simulink library "lib_EMachine_2017a"  (R2017b)
settings: Solver=VariableStepAuto  StartTime=0.0  StopTime=10.0  RelTol=1e-3
undefined symbols (not defined in the file): EngineTorqueReal, mot, motor_Trq, t_amb, time, tloop
libraries: simulink x5, autolibmappedmotor x3
(part 3 of 3)

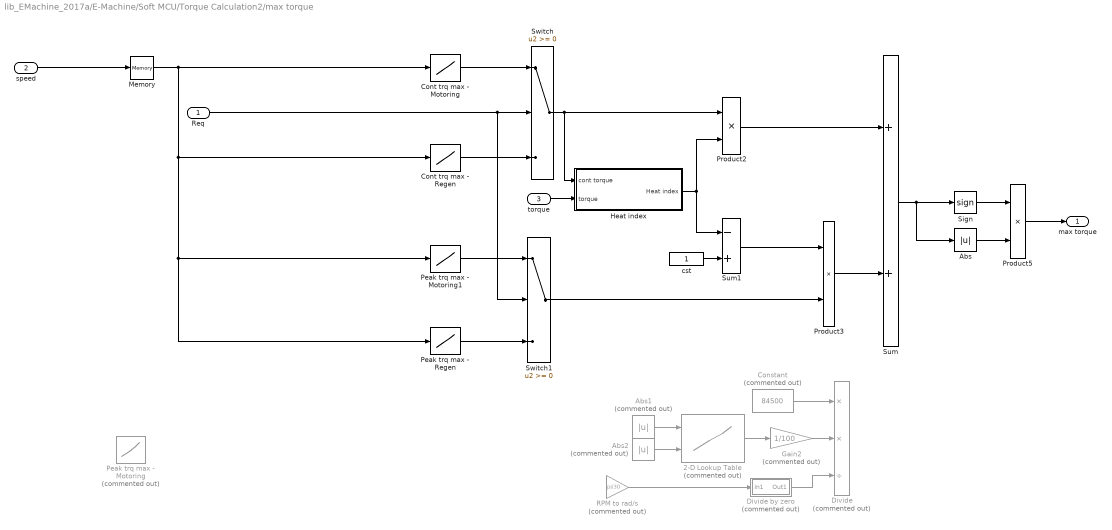
== system lib_EMachine_2017a/E-Machine/Soft MCU/Torque Calculation2/max torque  ==
  Req : Inport
  speed : Inport  Port=2
  torque : Inport  Port=3
  2-D Lookup Table : Lookup_n-D  Commented=on  BreakpointsForDimension1=mot.plant.init.eff_trq.idx2_trq  BreakpointsForDimension2=mot.plant.init.eff_trq.idx1_spd  Table=mot.plant.init.eff_trq.map  InternalRulePriority=Speed  RndMeth=Simplest  InputSameDT=on
  Abs : Abs  SaturateOnIntegerOverflow=on
  Abs1 : Abs  Commented=on
  Abs2 : Abs  Commented=on
  Constant : Constant  Commented=on  Value=84500
  Cont trq max - Motoring : Lookup  InputValues=mot.plant.init.motor.trq_cont.idx1_spd  Table=mot.plant.init.motor.trq_cont.map  LookUpMeth=Interpolation-Use End Values  SaturateOnIntegerOverflow=on
  Cont trq max - Regen : Lookup  InputValues=mot.plant.init.regen.trq_cont.idx1_spd  Table=mot.plant.init.regen.trq_cont.map  LookUpMeth=Interpolation-Use End Values  SaturateOnIntegerOverflow=on
  Divide : Product  Commented=on  Inputs=**/
  Divide by zero : Subsystem  Commented=on
  Gain2 : Gain  Commented=on  Gain=1/100
  Heat index : Subsystem
  Memory : Memory
  Peak trq max - Motoring : Lookup  Commented=on  InputValues=mot.plant.init.regen.trq_max.idx1_spd  Table=mot.plant.init.motor.trq_max.map  LookUpMeth=Interpolation-Use End Values  SaturateOnIntegerOverflow=on
  Peak trq max - Motoring1 : Lookup  InputValues=mot.plant.init.regen.trq_max.idx1_spd  Table=mot.plant.init.motor.trq_max.map  LookUpMeth=Interpolation-Use End Values  SaturateOnIntegerOverflow=on
  Peak trq max - Regen : Lookup  InputValues=mot.plant.init.regen.trq_max.idx1_spd  Table=mot.plant.init.regen.trq_max.map  LookUpMeth=Interpolation-Use End Values  SaturateOnIntegerOverflow=on
  Product2 : Product  SaturateOnIntegerOverflow=on  InputSameDT=on  OutDataTypeStr=Inherit: Same as first input
  Product3 : Product  SaturateOnIntegerOverflow=on  InputSameDT=on  OutDataTypeStr=Inherit: Same as first input
  Product5 : Product  SaturateOnIntegerOverflow=on  InputSameDT=on  OutDataTypeStr=Inherit: Same as first input
  RPM to rad/s : Gain  Commented=on  Gain=pi/30
  Sign : Signum
  Sum : Sum  SaturateOnIntegerOverflow=on  InputSameDT=on  OutDataTypeStr=Inherit: Same as first input
  Sum1 : Sum  Inputs=-+  SaturateOnIntegerOverflow=on  InputSameDT=on  OutDataTypeStr=Inherit: Same as first input
  Switch : Switch  SaturateOnIntegerOverflow=on
  Switch1 : Switch  SaturateOnIntegerOverflow=on
  cst : Constant
  max torque : Outport
  wires:
  Peak trq max - Motoring1/1 -> Switch1/1
  Divide by zero/1(Out1) -> Divide/3
  Req/1 -> Switch1/2, Switch/2
  Gain2/1 -> Divide/2
  2-D Lookup Table/1 -> Gain2/1
  Abs1/1 -> 2-D Lookup Table/1
  Abs2/1 -> 2-D Lookup Table/2
  RPM to rad/s/1 -> Divide by zero/1(In1)
  Constant/1 -> Divide/1
  speed/1 -> Memory/1
  Memory/1 -> Peak trq max - Regen/1, Peak trq max - Motoring1/1, Cont trq max - Regen/1, Cont trq max - Motoring/1
  Sign/1 -> Product5/1
  Product5/1 -> max torque/1
  Sum/1 -> Sign/1, Abs/1
  Abs/1 -> Product5/2
  torque/1 -> Heat index/2(torque)
  Cont trq max - Motoring/1 -> Switch/1
  Cont trq max - Regen/1 -> Switch/3
  Peak trq max - Regen/1 -> Switch1/3
  Switch/1 -> Product2/1, Heat index/1(cont torque)
  Switch1/1 -> Product3/2
  Product2/1 -> Sum/1
  Sum1/1 -> Product3/1
  Product3/1 -> Sum/2
  cst/1 -> Sum1/2
  Heat index/1(Heat index) -> Sum1/1, Product2/2

== system lib_EMachine_2017a/E-Machine/Soft MCU/Torque Calculation3/Subsystem ==
  In1 : Inport
  In2 : Inport  Port=2
  In3 : Inport  Port=3
  Switch : Switch  Criteria=u2 > Threshold  ZeroCross=off
  Torq : Outport
  wires:
  Switch/1 -> Torq/1
  In1/1 -> Switch/1
  In3/1 -> Switch/3
  In2/1 -> Switch/2

== system lib_EMachine_2017a/E-Machine/Soft MCU/Torque Calculation3/Subsystem1 ==
  In1 : Inport
  In2 : Inport  Port=2
  In3 : Inport  Port=3
  Switch : Switch  Criteria=u2 > Threshold  ZeroCross=off
  Current : Outport
  wires:
  In2/1 -> Switch/2
  In3/1 -> Switch/3
  In1/1 -> Switch/1
  Switch/1 -> Current/1

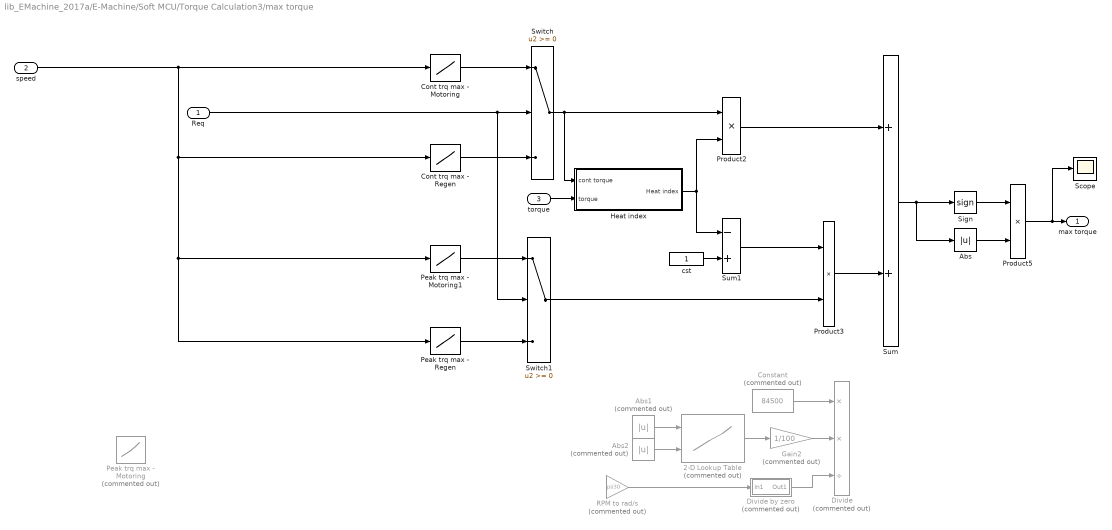
== system lib_EMachine_2017a/E-Machine/Soft MCU/Torque Calculation3/max torque  ==
  Req : Inport
  speed : Inport  Port=2
  torque : Inport  Port=3
  2-D Lookup Table : Lookup_n-D  Commented=on  BreakpointsForDimension1=mot.plant.init.eff_trq.idx2_trq  BreakpointsForDimension2=mot.plant.init.eff_trq.idx1_spd  Table=mot.plant.init.eff_trq.map  InternalRulePriority=Speed  RndMeth=Simplest  InputSameDT=on
  Abs : Abs  ZeroCross=off  SaturateOnIntegerOverflow=on
  Abs1 : Abs  Commented=on
  Abs2 : Abs  Commented=on
  Constant : Constant  Commented=on  Value=84500
  Cont trq max - Motoring : Lookup  InputValues=mot.plant.init.motor.trq_cont.idx1_spd  Table=mot.plant.init.motor.trq_cont.map  LookUpMeth=Interpolation-Use End Values  SaturateOnIntegerOverflow=on
  Cont trq max - Regen : Lookup  InputValues=mot.plant.init.regen.trq_cont.idx1_spd  Table=mot.plant.init.regen.trq_cont.map  LookUpMeth=Interpolation-Use End Values  SaturateOnIntegerOverflow=on
  Divide : Product  Commented=on  Inputs=**/
  Divide by zero : Subsystem  Commented=on
  Gain2 : Gain  Commented=on  Gain=1/100
  Heat index : Subsystem
  Peak trq max - Motoring : Lookup  Commented=on  InputValues=mot.plant.init.regen.trq_max.idx1_spd  Table=mot.plant.init.motor.trq_max.map  LookUpMeth=Interpolation-Use End Values  SaturateOnIntegerOverflow=on
  Peak trq max - Motoring1 : Lookup  InputValues=mot.plant.init.regen.trq_max.idx1_spd  Table=mot.plant.init.motor.trq_max.map  LookUpMeth=Interpolation-Use End Values  SaturateOnIntegerOverflow=on
  Peak trq max - Regen : Lookup  InputValues=mot.plant.init.regen.trq_max.idx1_spd  Table=mot.plant.init.regen.trq_max.map  LookUpMeth=Interpolation-Use End Values  SaturateOnIntegerOverflow=on
  Product2 : Product  SaturateOnIntegerOverflow=on  InputSameDT=on  OutDataTypeStr=Inherit: Same as first input
  Product3 : Product  SaturateOnIntegerOverflow=on  InputSameDT=on  OutDataTypeStr=Inherit: Same as first input
  Product5 : Product  SaturateOnIntegerOverflow=on  InputSameDT=on  OutDataTypeStr=Inherit: Same as first input
  RPM to rad/s : Gain  Commented=on  Gain=pi/30
  Scope : Scope
  Sign : Signum  ZeroCross=off
  Sum : Sum  SaturateOnIntegerOverflow=on  InputSameDT=on  OutDataTypeStr=Inherit: Same as first input
  Sum1 : Sum  Inputs=-+  SaturateOnIntegerOverflow=on  InputSameDT=on  OutDataTypeStr=Inherit: Same as first input
  Switch : Switch  SaturateOnIntegerOverflow=on
  Switch1 : Switch  SaturateOnIntegerOverflow=on
  cst : Constant
  max torque : Outport
  wires:
  Peak trq max - Motoring1/1 -> Switch1/1
  Divide by zero/1(Out1) -> Divide/3
  Req/1 -> Switch1/2, Switch/2
  Gain2/1 -> Divide/2
  2-D Lookup Table/1 -> Gain2/1
  Abs1/1 -> 2-D Lookup Table/1
  Abs2/1 -> 2-D Lookup Table/2
  RPM to rad/s/1 -> Divide by zero/1(In1)
  Constant/1 -> Divide/1
  speed/1 -> Peak trq max - Regen/1, Peak trq max - Motoring1/1, Cont trq max - Regen/1, Cont trq max - Motoring/1
  Sign/1 -> Product5/1
  Product5/1 -> max torque/1, Scope/1
  Sum/1 -> Sign/1, Abs/1
  Abs/1 -> Product5/2
  torque/1 -> Heat index/2(torque)
  Cont trq max - Motoring/1 -> Switch/1
  Cont trq max - Regen/1 -> Switch/3
  Peak trq max - Regen/1 -> Switch1/3
  Switch/1 -> Product2/1, Heat index/1(cont torque)
  Switch1/1 -> Product3/2
  Product2/1 -> Sum/1
  Sum1/1 -> Product3/1
  Product3/1 -> Sum/2
  cst/1 -> Sum1/2
  Heat index/1(Heat index) -> Sum1/1, Product2/2

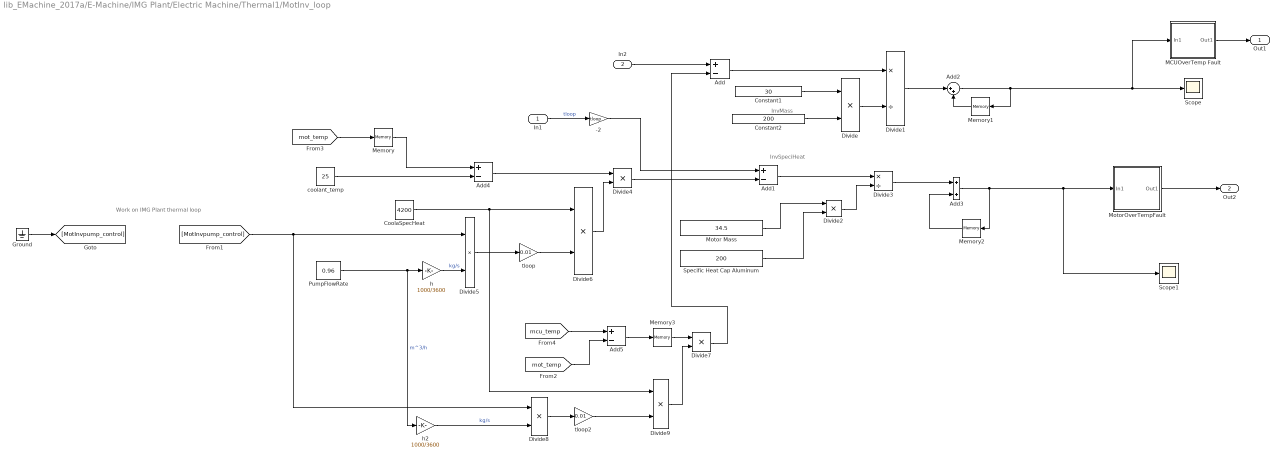
== system lib_EMachine_2017a/E-Machine/IMG Plant/Electric Machine/Thermal1/MotInv_loop ==
  note: InvSpeciHeat
  note: InvMass
  note: Work on IMG Plant thermal loop
  In1 : Inport
  In2 : Inport  Port=2
  -2 : Gain  Gain=tloop
  Add{,1,4..5} (4 alike) : Sum  Inputs=+-
  Add2 : Sum  Inputs=|++
  Add3 : Sum
  Constant1 : Constant  Value=30
  Constant2 : Constant  Value=200
  CoolaSpecHeat : Constant  Value=4200
  Divide{,2,4..9} (8 alike) : Product  Inputs=**
  Divide1 : Product  Inputs=*/
  Divide3 : Product  Inputs=*/
  Ground : Ground
  MCUOverTemp Fault : Subsystem
  Memory : Memory
  Memory1 : Memory  InitialCondition=25
  Memory2 : Memory  InitialCondition=25
  Memory3 : Memory
  Motor Mass : Constant  Value=34.5
  MotorOverTempFault : Subsystem
  PumpFlowRate : Constant  Value=0.96
  Scope : Scope
  Scope1 : Scope
  Specific Heat Cap Aluminum : Constant  Value=200
  coolant_temp : Constant  Value=25
  h : Gain  Gain=1000/3600
  h2 : Gain  Gain=1000/3600
  tloop : Gain  Gain=0.01
  tloop2 : Gain  Gain=0.01
  Out1 : Outport
  Out2 : Outport  Port=2
  wires:
  Ground/1 -> [MotInvpump_control]
  Memory/1 -> Add4/1
  Add1/1 -> Divide3/1
  Memory1/1 -> Add2/2
  coolant_temp/1 -> Add4/2
  Divide/1 -> Divide1/2
  Specific Heat Cap Aluminum/1 -> Divide2/2
  Constant1/1 -> Divide/1
  Add/1 -> Divide1/1
  Memory2/1 -> Add3/2
  Add4/1 -> Divide4/1
  Add3/1 -> Scope1/1, MotorOverTempFault/1(In1), Memory2/1
  Divide6/1 -> Divide4/2
  Divide3/1 -> Add3/1
  Divide5/1 -> tloop/1
  Add2/1 -> MCUOverTemp Fault/1(In1), Scope/1, Memory1/1
  Divide2/1 -> Divide3/2
  Constant2/1 -> Divide/2
  Motor Mass/1 -> Divide2/1
  Divide1/1 -> Add2/1
  Divide7/1 -> Add/2
  h/1 -> Divide5/2  "kg/s"
  tloop/1 -> Divide6/2
  CoolaSpecHeat/1 -> Divide6/1, Divide9/1
  PumpFlowRate/1 -> h/1, h2/1  "m^3/h"
  h2/1 -> Divide8/2  "kg/s"
  Divide9/1 -> Divide7/2
  Divide8/1 -> tloop2/1
  tloop2/1 -> Divide9/2
  Divide4/1 -> Add1/2
  Add5/1 -> Memory3/1
  Memory3/1 -> Divide7/1
  MCUOverTemp Fault/1(Out1) -> Out1/1
  MotorOverTempFault/1(Out1) -> Out2/1
  [mot_temp] -> Memory/1
  [mcu_temp] -> Add5/1
  [mot_temp] -> Add5/2
  In1/1 -> -2/1  "tloop"
  In2/1 -> Add/1
  -2/1 -> Add1/1
  [MotInvpump_control] -> Divide5/1, Divide8/1

== system lib_EMachine_2017a/E-Machine/IMG Plant/Electric Machine/Thermal1/Motor Thermal ==
  In1 : Inport
  Add1 : Sum  Inputs=+-
  Add2 : Sum
  Divide : Product  Inputs=*/
  Lower Limit : Subsystem  mask{Lolimit=t_amb+20}
      mask prompts: Lolimit "Lower Limit"
  Memory1 : Memory
  Motor Mass : Constant  Value=mot.plant.init.motor_mass
  Product : Product  RndMeth=Zero
  "Pump " : Constant  Value=0
  Specific Heat Cap Aluminum : Constant  Value=mot.plant.init.specific_heat
  tloop : Gain  Gain=tloop
  Out1 : Outport
  wires:
  Specific Heat Cap Aluminum/1 -> Product/2  "J/kg*K"
  Product/1 -> Divide/2
  Memory1/1 -> Add2/2
  Add2/1 -> Lower Limit/1(In1)
  Lower Limit/1(Out1) -> Out1/1, Memory1/1
  Divide/1 -> Add2/1
  tloop/1 -> Divide/1  "J"
  Motor Mass/1 -> Product/1  "kg"
  "Pump "/1 -> Add1/2
  In1/1 -> Add1/1
  Add1/1 -> tloop/1

== system lib_EMachine_2017a/E-Machine/IMG Plant/Electric Machine/Torque Calculation1/max torque  ==
  cmd : Inport
  speed : Inport  Port=2
  Memory : Memory
  Peak trq max - Motoring : Lookup  InputValues=mot.plant.init.regen.trq_max.idx1_spd  Table=mot.plant.init.motor.trq_max.map  LookUpMeth=Interpolation-Use End Values  SaturateOnIntegerOverflow=on
  Peak trq max - Regen : Lookup  InputValues=mot.plant.init.regen.trq_max.idx1_spd  Table=mot.plant.init.regen.trq_max.map  LookUpMeth=Interpolation-Use End Values  SaturateOnIntegerOverflow=on
  Switch1 : Switch  SaturateOnIntegerOverflow=on
  rad/s  to RPM : Gain  Gain=30/pi
  max torque : Outport
  wires:
  Peak trq max - Motoring/1 -> Switch1/1
  speed/1 -> rad/s  to RPM/1
  cmd/1 -> Switch1/2
  Switch1/1 -> max torque/1
  Memory/1 -> Peak trq max - Motoring/1, Peak trq max - Regen/1
  rad/s  to RPM/1 -> Memory/1
  Peak trq max - Regen/1 -> Switch1/3

== system lib_EMachine_2017a/E-Machine/IMG Plant2/Thermal/Motor Thermal/Lower Limit ==
  In1 : Inport
  Constant3 : Constant  Value=Lolimit
  MinMax : MinMax  Function=max  Inputs=2
  Out1 : Outport
  wires:
  In1/1 -> MinMax/1
  Constant3/1 -> MinMax/2
  MinMax/1 -> Out1/1

== system lib_EMachine_2017a/E-Machine/IMG Plant2/Thermal1/MotInv_loop/MCUOverTemp Fault ==
  In1 : Inport
  Gain : Gain  Gain=3
  Switch : Switch  Threshold=1
  Out1 : Outport
  wires:
  In1/1 -> Switch/3, Gain/1
  [MCUOverTemp] -> Switch/2
  Gain/1 -> Switch/1
  Switch/1 -> Out1/1

== system lib_EMachine_2017a/E-Machine/IMG Plant2/Thermal1/MotInv_loop/MotorOverTempFault ==
  In1 : Inport
  Gain : Gain  Gain=2
  Switch1 : Switch  Threshold=1
  Out1 : Outport
  wires:
  In1/1 -> Gain/1, Switch1/3
  [MotOverTemp] -> Switch1/2
  Gain/1 -> Switch1/1
  Switch1/1 -> Out1/1

== system lib_EMachine_2017a/E-Machine/IMG Plant2/Thermal1/Motor Thermal/Lower Limit ==
  In1 : Inport
  Constant3 : Constant  Value=Lolimit
  MinMax : MinMax  Function=max  Inputs=2
  Out1 : Outport
  wires:
  In1/1 -> MinMax/1
  Constant3/1 -> MinMax/2
  MinMax/1 -> Out1/1

== system lib_EMachine_2017a/E-Machine/Soft MCU/Torque Calculation1/max torque /Divide by zero ==
  In1 : Inport
  Compare To Constant : simulink/Logic and Bit Operations/Compare To Constant  relop===  const=0  OutDataTypeStr=boolean
  Constant1 : Constant
  Switch2 : Switch  Criteria=u2 > Threshold
  Out1 : Outport
  wires:
  Switch2/1 -> Out1/1
  In1/1 -> Compare To Constant/1, Switch2/3
  Compare To Constant/1 -> Switch2/2
  Constant1/1 -> Switch2/1

== system lib_EMachine_2017a/E-Machine/Soft MCU/Torque Calculation1/max torque /Heat index ==
  note: Heat index calculation
  cont torque : Inport
  torque : Inport  Port=2
  Abs : Abs  SaturateOnIntegerOverflow=on
  Divide : Subsystem  mask(Divide){}
      mask Display: disp('Divide')
  Heat Energy Factor : Integrator  InitialCondition=-0.3  LimitOutput=on  UpperSaturationLimit=1  LowerSaturationLimit=-0.3
  Heating Constant : Gain  Gain=0.3/mot.plant.init.t_max_trq  SaturateOnIntegerOverflow=on  OutDataTypeStr=Inherit: Same as input  ParamDataTypeStr=Inherit: Same as input
  Saturation : Saturate  UpperLimit=1  LowerLimit=0
  Sum : Sum  Inputs=+-  SaturateOnIntegerOverflow=on  InputSameDT=on  OutDataTypeStr=Inherit: Same as first input
  motor inertia (Nms^2\rad)5 : Constant
  Heat index : Outport
  wires:
  torque/1 -> Divide/1(numerator)
  Heat Energy Factor/1 -> Saturation/1
  Heating Constant/1 -> Heat Energy Factor/1
  Sum/1 -> Heating Constant/1
  Divide/1(quotient) -> Abs/1
  motor inertia (Nms^2\rad)5/1 -> Sum/2
  Saturation/1 -> Heat index/1
  Abs/1 -> Sum/1
  cont torque/1 -> Divide/2(denominator)

== system lib_EMachine_2017a/E-Machine/Soft MCU/Torque Calculation2/max torque /Divide by zero ==
  In1 : Inport
  Compare To Constant : simulink/Logic and Bit Operations/Compare To Constant  relop===  const=0  OutDataTypeStr=boolean
  Constant1 : Constant
  Switch2 : Switch  Criteria=u2 > Threshold
  Out1 : Outport
  wires:
  Switch2/1 -> Out1/1
  In1/1 -> Compare To Constant/1, Switch2/3
  Compare To Constant/1 -> Switch2/2
  Constant1/1 -> Switch2/1

== system lib_EMachine_2017a/E-Machine/Soft MCU/Torque Calculation2/max torque /Heat index ==
  note: Heat index calculation
  cont torque : Inport
  torque : Inport  Port=2
  Abs : Abs  SaturateOnIntegerOverflow=on
  Divide : Subsystem  mask(Divide){}
      mask Display: disp('Divide')
  Heat Energy Factor : Integrator  InitialCondition=-0.3  LimitOutput=on  UpperSaturationLimit=1  LowerSaturationLimit=-0.3
  Heating Constant : Gain  Gain=0.3/mot.plant.init.t_max_trq  SaturateOnIntegerOverflow=on  OutDataTypeStr=Inherit: Same as input  ParamDataTypeStr=Inherit: Same as input
  Saturation : Saturate  UpperLimit=1  LowerLimit=0
  Sum : Sum  Inputs=+-  SaturateOnIntegerOverflow=on  InputSameDT=on  OutDataTypeStr=Inherit: Same as first input
  motor inertia (Nms^2\rad)5 : Constant
  Heat index : Outport
  wires:
  torque/1 -> Divide/1(numerator)
  Heat Energy Factor/1 -> Saturation/1
  Heating Constant/1 -> Heat Energy Factor/1
  Sum/1 -> Heating Constant/1
  Divide/1(quotient) -> Abs/1
  motor inertia (Nms^2\rad)5/1 -> Sum/2
  Saturation/1 -> Heat index/1
  Abs/1 -> Sum/1
  cont torque/1 -> Divide/2(denominator)

== system lib_EMachine_2017a/E-Machine/Soft MCU/Torque Calculation3/max torque /Divide by zero ==
  In1 : Inport
  Compare To Constant : simulink/Logic and Bit Operations/Compare To Constant  relop===  const=0  OutDataTypeStr=boolean
  Constant1 : Constant
  Switch2 : Switch  Criteria=u2 > Threshold
  Out1 : Outport
  wires:
  Switch2/1 -> Out1/1
  In1/1 -> Compare To Constant/1, Switch2/3
  Compare To Constant/1 -> Switch2/2
  Constant1/1 -> Switch2/1

== system lib_EMachine_2017a/E-Machine/Soft MCU/Torque Calculation3/max torque /Heat index ==
  note: Heat index calculation
  cont torque : Inport
  torque : Inport  Port=2
  Abs : Abs  ZeroCross=off  SaturateOnIntegerOverflow=on
  Divide : Subsystem  mask(Divide){}
      mask Display: disp('Divide')
  Heat Energy Factor : Integrator  InitialCondition=-0.3  LimitOutput=on  UpperSaturationLimit=1  LowerSaturationLimit=-0.3  ZeroCross=off
  Heating Constant : Gain  Gain=0.3/mot.plant.init.t_max_trq  SaturateOnIntegerOverflow=on  OutDataTypeStr=Inherit: Same as input  ParamDataTypeStr=Inherit: Same as input
  Saturation : Saturate  UpperLimit=1  LowerLimit=0  ZeroCross=off
  Sum : Sum  Inputs=+-  SaturateOnIntegerOverflow=on  InputSameDT=on  OutDataTypeStr=Inherit: Same as first input
  motor inertia (Nms^2\rad)5 : Constant
  Heat index : Outport
  wires:
  torque/1 -> Divide/1(numerator)
  Heat Energy Factor/1 -> Saturation/1
  Heating Constant/1 -> Heat Energy Factor/1
  Sum/1 -> Heating Constant/1
  Divide/1(quotient) -> Abs/1
  motor inertia (Nms^2\rad)5/1 -> Sum/2
  Saturation/1 -> Heat index/1
  Abs/1 -> Sum/1
  cont torque/1 -> Divide/2(denominator)

== system lib_EMachine_2017a/E-Machine/IMG Plant/Electric Machine/Thermal1/MotInv_loop/MCUOverTemp Fault ==
  In1 : Inport
  Gain : Gain  Gain=3
  Switch : Switch  Threshold=1
  Out1 : Outport
  wires:
  In1/1 -> Switch/3, Gain/1
  [MCUOverTemp] -> Switch/2
  Gain/1 -> Switch/1
  Switch/1 -> Out1/1

== system lib_EMachine_2017a/E-Machine/IMG Plant/Electric Machine/Thermal1/MotInv_loop/MotorOverTempFault ==
  In1 : Inport
  Gain : Gain  Gain=2
  Memory : Memory
  Switch1 : Switch  Threshold=1
  Out1 : Outport
  wires:
  Memory/1 -> Gain/1
  In1/1 -> Memory/1, Switch1/3
  [MotOverTemp] -> Switch1/2
  Gain/1 -> Switch1/1
  Switch1/1 -> Out1/1

== system lib_EMachine_2017a/E-Machine/IMG Plant/Electric Machine/Thermal1/Motor Thermal/Lower Limit ==
  In1 : Inport
  Constant3 : Constant  Value=Lolimit
  MinMax : MinMax  Function=max  Inputs=2
  Out1 : Outport
  wires:
  In1/1 -> MinMax/1
  Constant3/1 -> MinMax/2
  MinMax/1 -> Out1/1

== system lib_EMachine_2017a/E-Machine/Soft MCU/Torque Calculation1/max torque /Heat index/Divide ==
  note: Take care of
      | division by 0
  numerator : Inport
  denominator : Inport  Port=2
  Fcn : Fcn  Expr=u[1] / ( u[2] + eps*(u[2]==0) )
  Mux : Mux  Inputs=2
  quotient : Outport
  wires:
  Mux/1 -> Fcn/1
  numerator/1 -> Mux/1
  Fcn/1 -> quotient/1
  denominator/1 -> Mux/2

== system lib_EMachine_2017a/E-Machine/Soft MCU/Torque Calculation2/max torque /Heat index/Divide ==
  note: Take care of
      | division by 0
  numerator : Inport
  denominator : Inport  Port=2
  Fcn : Fcn  Expr=u[1] / ( u[2] + eps*(u[2]==0) )
  Mux : Mux  Inputs=2
  quotient : Outport
  wires:
  Mux/1 -> Fcn/1
  numerator/1 -> Mux/1
  Fcn/1 -> quotient/1
  denominator/1 -> Mux/2

== system lib_EMachine_2017a/E-Machine/Soft MCU/Torque Calculation3/max torque /Heat index/Divide ==
  note: Take care of
      | division by 0
  numerator : Inport
  denominator : Inport  Port=2
  Fcn : Fcn  Expr=u[1] / ( u[2] + eps*(u[2]==0) )
  Mux : Mux  Inputs=2
  quotient : Outport
  wires:
  Mux/1 -> Fcn/1
  numerator/1 -> Mux/1
  Fcn/1 -> quotient/1
  denominator/1 -> Mux/2

== matlab function lib_EMachine_2017a/E-Machine/Soft MCU/diff_INV_state ==
  data: u input; y output
function y = fcn(u)
if(u == 3) %when inverter is in standby state
    y = 0;
elseif(u == 8) %when inverter is in torque control state
    y = 1;
elseif(u==14) %when invertor is in error state
    y = 2;
else
    y = 0;
end

== matlab function lib_EMachine_2017a/E-Machine/Soft MCU/diff_INV_state1 ==
  data: u input; y output
function y = fcn(u)
if(u == 0) %when inverter is in standby state
    y = 0;
elseif(u == 1) %when inverter is in torque control state
    y = 1;
elseif(u==2) %when invertor is in error state
    y = 0;
else
    y = 0;
end
